simulink model "Animation_Try_1"  (R2025a)
settings: Solver=VariableStepAuto  StartTime=0.0  StopTime=4000  RelTol=1e-3
libraries: aerolibanim x1, aerolibatmos2 x1, sharedutil x1
settings Model: Creator=shauryagupta  LastModifiedBy=shauryagupta

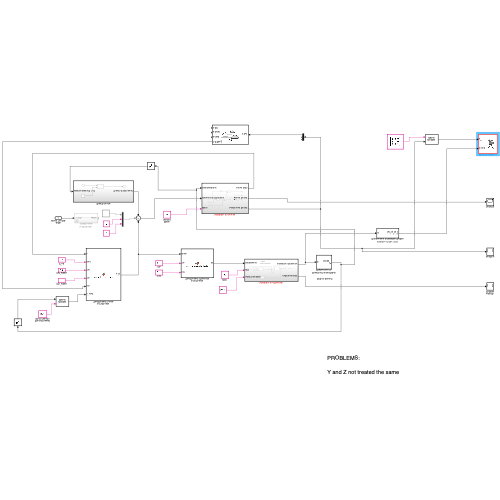
[thumbnail: Simulink's stored preview of the top-level diagram]
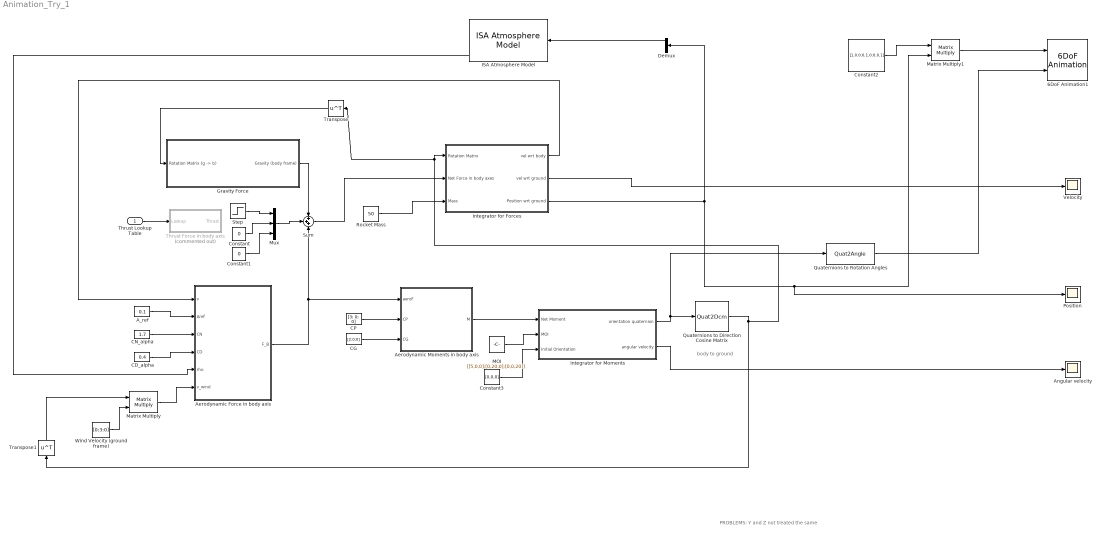
== system Animation_Try_1 ==
  note: PROBLEMS:
      |
      | Y and Z not treated the same
  note: body to ground
  Thrust Lookup Table : Inport
  6DoF Animation1 : aerolibanim/6DoF Animation  u1=[0 4000 -2000 2000 -5000 -3000]  u2=0.2  u3=100  u4=[4000 0 -5000]  u5=Fly alongside  u6=[2000 500 -3150]  u7=7  u8=on
  A_ref : Constant  Value=0.1
  Aerodynamic Force in body axis : MATLAB Function  TreatAsAtomicUnit=on
  Aerodynamic Moments in body axis : MATLAB Function  TreatAsAtomicUnit=on
  Angular velocity : Scope
      settings: ActiveDisplayYMinimum=-0.27819491647133165  ActiveDisplayYMaximum=0.29194633809320797  DataLoggingVariableName=ScopeData2
  CD_alpha : Constant  Value=0.4
  CG : Constant  Value=[2;0;0]  VectorParams1D=off
  CN_alpha : Constant  Value=1.7
  CP : Constant  Value=[3; 0; 0]
  Constant : Constant  Value=0
  Constant1 : Constant  Value=0
  Constant2 : Constant  Value=[1,0,0;0,1,0;0,0,1]
  Constant3 : Constant  Value=[0,0,0]
  Demux : Demux  Outputs=3
  Gravity Force : Subsystem
  ISA Atmosphere Model : aerolibatmos2/ISA Atmosphere Model  useExtended=off  action=None  custom=off  viscosityOut=off  g=9.80665  gamma=1.4  R=287.0531  L=0.0065  h_trop=11000  h_strat=20000  rho0=1.225  P0=101325  T0=288.15  h0=0  S=110.4  Tref=273.15  muref=1.716e-5
  Integrator for Forces : Subsystem
  Integrator for Moments : Subsystem
  MOI : Constant  Value=[[5,0,0];[0,20,0];[0,0,20]]
  Matrix Multiply : Product  Multiplication=Matrix(*)
  Matrix Multiply1 : Product  Multiplication=Matrix(*)
  Mux : Mux  Inputs=3
  Position : Scope
      settings: ActiveDisplayYMinimum=-9371.1645521574628  ActiveDisplayYMaximum=6479.3379800634129
  "Quaternions to Direction Cosine Matrix " : Quat2Dcm
  Quaternions to Rotation Angles : Quat2Angle  rotationOrder=XYZ
      settings: AttributesFormatString=Rotation Order: %<rotationOrder>
  Rocket Mass : Constant  Value=50
  Step : Step  Time=5  Before=4000  After=0  SampleTime=0
  Sum : Sum  Inputs=+++
  "Thrust Force in body axis " : Subsystem  Commented=on
  Transpose : Math  Operator=transpose
  Transpose1 : Math  Operator=transpose
  Velocity : Scope
      settings: ActiveDisplayYMinimum=-64.707758735669429  ActiveDisplayYMaximum=349.31979200881909
  Wind Velocity (ground frame) : Constant  Value=[0;3;0]
  wires:
  Sum/1 -> Integrator for Forces/2("Net Force in body axes ")
  CP/1 -> Aerodynamic Moments in body axis/2(CP)
  Transpose/1 -> Gravity Force/1("Rotation Matrix (g -> b) ")
  Wind Velocity (ground frame)/1 -> Matrix Multiply/2
  Thrust Lookup Table/1 -> "Thrust Force in body axis "/1(Lookup)
  Integrator for Moments/1(orientation quaternion) -> Quaternions to Rotation Angles/1, "Quaternions to Direction Cosine Matrix "/1
  Gravity Force/1(Gravity (body frame)) -> Sum/1
  Constant/1 -> Mux/2
  "Quaternions to Direction Cosine Matrix "/1 -> Transpose/1, Integrator for Forces/1(Rotation Matrix), Transpose1/1
  Rocket Mass/1 -> Integrator for Forces/3(Mass)
  Transpose1/1 -> Matrix Multiply/1
  Step/1 -> Mux/1
  Demux/1 -> ISA Atmosphere Model/1
  A_ref/1 -> Aerodynamic Force in body axis/2(Aref)
  Aerodynamic Force in body axis/1(F_B) -> Sum/3, Aerodynamic Moments in body axis/1(aeroF)
  Integrator for Moments/2(angular velocity) -> Angular velocity/1
  Constant1/1 -> Mux/3
  Integrator for Forces/2(vel wrt ground) -> Velocity/1
  Aerodynamic Moments in body axis/1(M) -> Integrator for Moments/1(Net Moment)
  CN_alpha/1 -> Aerodynamic Force in body axis/3(CN)
  MOI/1 -> Integrator for Moments/2(MOI)
  CG/1 -> Aerodynamic Moments in body axis/3(CG)
  Matrix Multiply/1 -> Aerodynamic Force in body axis/6(v_wind)
  CD_alpha/1 -> Aerodynamic Force in body axis/4(CD)
  Integrator for Forces/3(Position wrt ground) -> Matrix Multiply1/2, Position/1, Demux/1
  Mux/1 -> Sum/2
  Integrator for Forces/1(vel wrt body) -> Aerodynamic Force in body axis/1(v)
  ISA Atmosphere Model/4 -> Aerodynamic Force in body axis/5(rho)
  Quaternions to Rotation Angles/1 -> 6DoF Animation1/2
  Matrix Multiply1/1 -> 6DoF Animation1/1
  Constant2/1 -> Matrix Multiply1/1
  Constant3/1 -> Integrator for Moments/3(Initial Orientation)

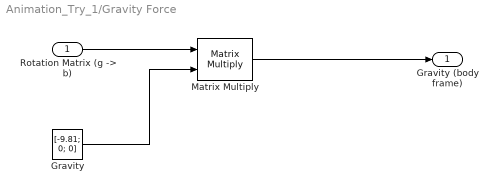
== system Animation_Try_1/Gravity Force ==
  "Rotation Matrix (g -> b) " : Inport
  Gravity : Constant  Value=[-9.81; 0; 0]
  Matrix Multiply : Product  Multiplication=Matrix(*)
  Gravity (body frame) : Outport
  wires:
  "Rotation Matrix (g -> b) "/1 -> Matrix Multiply/1
  Gravity/1 -> Matrix Multiply/2
  Matrix Multiply/1 -> Gravity (body frame)/1

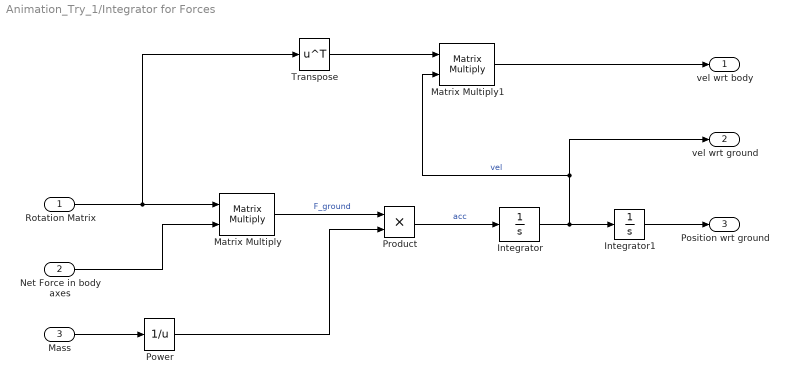
== system Animation_Try_1/Integrator for Forces ==
  Rotation Matrix : Inport
  "Net Force in body axes " : Inport  Port=2
  Mass : Inport  Port=3
  Integrator : Integrator  InitialCondition=[0; 0; 0]
  Integrator1 : Integrator  InitialCondition=[0; 0; 0]
  Matrix Multiply : Product  Multiplication=Matrix(*)
  Matrix Multiply1 : Product  Multiplication=Matrix(*)
  Power : Math  Operator=reciprocal
  Product : Product
  Transpose : Math  Operator=transpose
  vel wrt body : Outport
  vel wrt ground : Outport  Port=2
  Position wrt ground : Outport  Port=3
  wires:
  Rotation Matrix/1 -> Transpose/1, Matrix Multiply/1
  "Net Force in body axes "/1 -> Matrix Multiply/2
  Mass/1 -> Power/1
  Matrix Multiply/1 -> Product/1  "F_ground"
  Power/1 -> Product/2
  Product/1 -> Integrator/1  "acc"
  Integrator/1 -> Matrix Multiply1/2, vel wrt ground/1, Integrator1/1  "vel"
  Integrator1/1 -> Position wrt ground/1
  Transpose/1 -> Matrix Multiply1/1
  Matrix Multiply1/1 -> vel wrt body/1

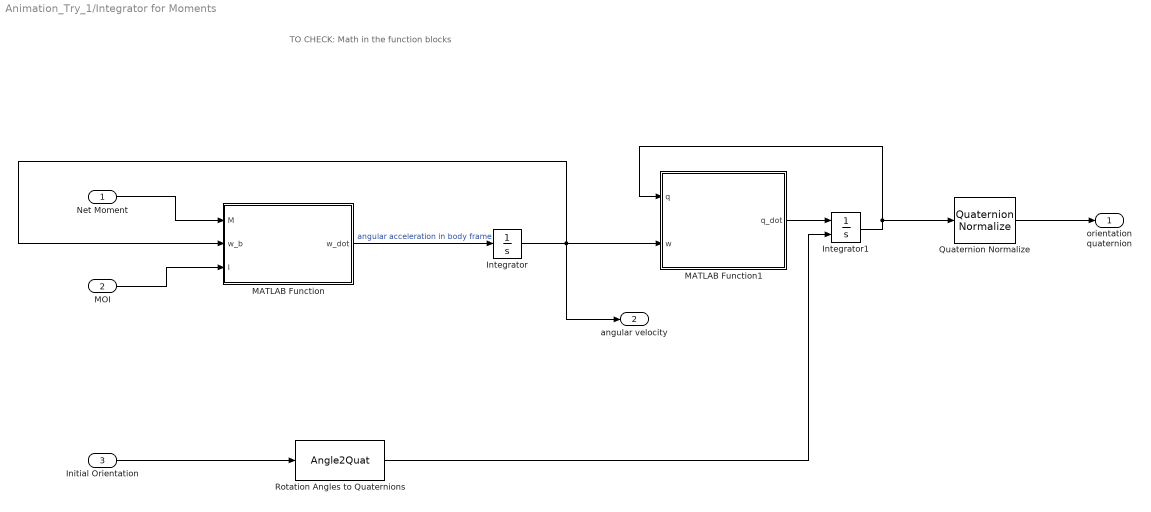
== system Animation_Try_1/Integrator for Moments ==
  note: TO CHECK:
      |
      | Math in the function blocks
  Net Moment : Inport
  MOI : Inport  Port=2
  Initial Orientation : Inport  Port=3
  Integrator : Integrator  InitialCondition=[0; 0; 0]
  Integrator1 : Integrator  InitialConditionSource=external  InitialCondition=[1; 0; 0; 0]  ContinuousStateAttributes='orientation'
  MATLAB Function : MATLAB Function  TreatAsAtomicUnit=on
  MATLAB Function1 : MATLAB Function  TreatAsAtomicUnit=on
  Quaternion Normalize : sharedutil/Quaternion Normalize  aMode=aMode
  Rotation Angles to Quaternions : Angle2Quat  rotationOrder=XYZ
      settings: AttributesFormatString=Rotation Order: %<rotationOrder>
  orientation quaternion : Outport
  angular velocity : Outport  Port=2
  wires:
  Net Moment/1 -> MATLAB Function/1(M)
  MOI/1 -> MATLAB Function/3(I)
  Integrator/1 -> MATLAB Function/2(w_b), MATLAB Function1/2(w), angular velocity/1
  MATLAB Function/1(w_dot) -> Integrator/1  "angular acceleration in body frame"
  MATLAB Function1/1(q_dot) -> Integrator1/1
  Integrator1/1 -> MATLAB Function1/1(q), Quaternion Normalize/1
  Quaternion Normalize/1 -> orientation quaternion/1
  Rotation Angles to Quaternions/1 -> Integrator1/2
  Initial Orientation/1 -> Rotation Angles to Quaternions/1

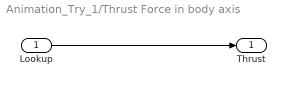
== system Animation_Try_1/Thrust Force in body axis  ==
  Lookup : Inport
  Thrust : Outport
  wires:
  Lookup/1 -> Thrust/1

== matlab function Animation_Try_1/Integrator for Moments/MATLAB Function ==
  data: M input; w_dot output; w_b input; I input
function w_dot = angular_vel(M, w_b, I)
%#codegen


angular_vel = I \ ( M - cross(w_b, I*w_b) );

w_dot = angular_vel;

if any(~isfinite(M))
    w_dot = [0;0;0];
    return
end

== matlab function Animation_Try_1/Aerodynamic Moments in body axis ==
  data: aeroF input; M output; CP input; CG input
function M = aero_moments_body(aeroF, CP, CG)
%#codegen
% CP, CG, Fb -> 3 X 1 vectors


r = CP - CG;

if norm(aeroF) < 1e-3
    M = [0; 0; 0];
else
    M = cross(r, aeroF);

end

== matlab function Animation_Try_1/Integrator for Moments/MATLAB Function1 ==
  data: q input; q_dot output; w input
function q_dot = quat_dot_from_omega(q, w)
% Inputs:
%   q : 4x1 quaternion [q0; q1; q2; q3]
%   w : 3x1 angular velocity [wx; wy; wz] (rad/s)
%
% Output:
%   q_dot : 4x1 quaternion derivative

wx = w(1);
wy = w(2);
wz = w(3);

Omega = [  0  -wx -wy -wz;
           wx   0  -wz  wy;
           wy   wz  0  -wx;
           wz  -wy  wx  0 ];

q_dot = 0.5 * Omega * q;
end

== matlab function Animation_Try_1/Aerodynamic Force in body axis ==
  data: v input; F_B output; Aref input; CN input; CD input; rho input; v_wind input
function F_B = aero_forces_body(v, Aref, CN, CD, rho, v_wind)
% ----------------------------------------------------
% Computes total aerodynamic force in BODY frame
%
% Inputs:
% vB   : 3x1 velocity vector in body frame [m/s]
% rho  : air density [kg/m^3]
% Aref : reference area [m^2]
% CN   : normal force coefficient
% CD   : drag coefficient
%
% Output:
% F_B  : 3x1 aerodynamic force vector in body frame [N]
% ----------------------------------------------------

% Unpack velocity

vB = v - v_wind;

vx = vB(1);
vy = vB(2);
vz = vB(3);


V = norm(vB);

% Guard against zero velocity
if V < 1e-3
    F_B = [0; 0; 0];
    return
end

% Dynamic pressure
q = 0.5 * rho * V^2;

% -------------------------
% Drag force (opposite wind)
% -------------------------
drag_dir = -vB / V;   % unit vector opposite rocket velocity
F_drag = CD * q * Aref * drag_dir;

F_normal = -CN * q * Aref * [0; vB(2); vB(3)] / V;

% -------------------------
% Total aerodynamic force
% -------------------------
F_B = F_drag + F_normal;

end
